simulink library "INT_APP_VD"  (R2016b)
settings: Solver=VariableStepAuto  StartTime=0.0  StopTime=10.0  RelTol=1e-3
settings Model: Creator=zhoutinglin  LastModifiedBy=zhoutinglin

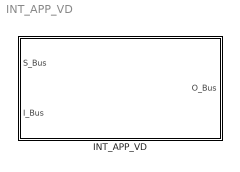
== system INT_APP_VD ==
  INT_APP_VD : Subsystem

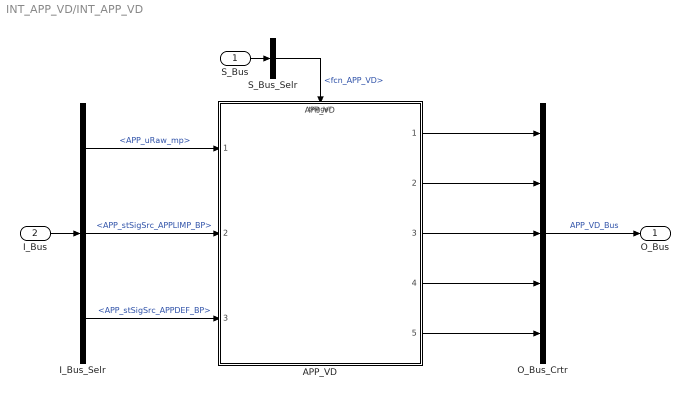
== system INT_APP_VD/INT_APP_VD ==
  S_Bus : Inport
  I_Bus : Inport  Port=2
  APP_VD : ModelReference  ModelNameDialog=APP_VD  SimulationMode=Normal  ModelReferenceVersion=1.35  TriggerPortName=function  TriggerPortTriggerType=function-call  TriggerPortStatesWhenEnabling=held
  I_Bus_Selr : BusSelector  OutputSignals=APP_uRaw_mp,APP_stSigSrc_APPLIMP_BP,APP_stSigSrc_APPDEF_BP
  O_Bus_Crtr : BusCreator  Inputs=5
  S_Bus_Selr : BusSelector  OutputSignals=fcn_APP_VD
  O_Bus : Outport
  wires:
  S_Bus_Selr/1 -> APP_VD/Trigger  "<fcn_APP_VD>"
  S_Bus/1 -> S_Bus_Selr/1
  I_Bus/1 -> I_Bus_Selr/1
  I_Bus_Selr/1 -> APP_VD/1  "<APP_uRaw_mp>"
  I_Bus_Selr/2 -> APP_VD/2  "<APP_stSigSrc_APPLIMP_BP>"
  I_Bus_Selr/3 -> APP_VD/3  "<APP_stSigSrc_APPDEF_BP>"
  O_Bus_Crtr/1 -> O_Bus/1  "APP_VD_Bus"
  APP_VD/1 -> O_Bus_Crtr/1
  APP_VD/2 -> O_Bus_Crtr/2
  APP_VD/3 -> O_Bus_Crtr/3
  APP_VD/4 -> O_Bus_Crtr/4
  APP_VD/5 -> O_Bus_Crtr/5
